simulink model "LQR1"  (R2020a)
settings: Solver=VariableStepAuto  StartTime=0.0  StopTime=300  RelTol=1e-3
values from neighbouring files (symbols this model uses):
  A = zeros(n_states)    [RIP.m]
  B = zeros(n_states,n_inputs)    [RIP.m]
  Ki = K_d_Int(:,1)    [RIP.m]
  Ks = K_d_Int(:,2:end)    [RIP.m]
  n_inputs = 1    [RIP.m]
  n_states = 4    [RIP.m]
  Ts = 1/200    (= 0.005)    [RIP.m]
libraries: dspsrcs4 x1
settings Model: Creator=user  LastModifiedBy=user

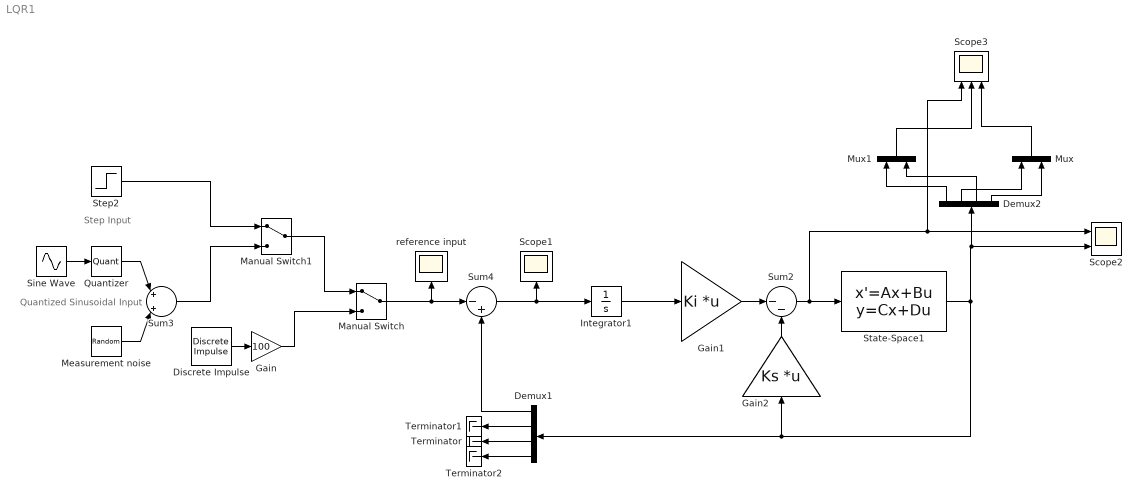
== system LQR1 ==
  note: Quantized Sinusoidal Input
  note: Step Input
  Demux1 : Demux
  Demux2 : Demux
  Discrete Impulse : dspsrcs4/Discrete  Impulse  Delay=0  SampleTime=0.01  FrameSample=1  OutputFrames=off  dataType=double  isSigned=on  wordLen=16  udDataType=sfix(16)  fracBitsMode=Best precision  numFracBits=15  OutDataTypeStr=double  LastOutDataTypeStr=double
  Gain : Gain  Gain=100
  Gain1 : Gain  Gain=Ki  Multiplication=Matrix(K*u)
  Gain2 : Gain  Gain=Ks  Multiplication=Matrix(K*u)
  Integrator1 : Integrator
  Manual Switch : ManualSwitch
  Manual Switch1 : ManualSwitch
  Measurement noise : RandomNumber  Variance=0.0000001  SampleTime=Ts
  Mux : Mux  Inputs=2
  Mux1 : Mux  Inputs=2
  Quantizer : Quantizer  QuantizationInterval=2^(-12)
  Scope1 : Scope
  Scope2 : Scope  NumInputPorts=2
  Scope3 : Scope  NumInputPorts=3
  Sine Wave : Sin  Amplitude=pi/4  Frequency=0.2  SampleTime=Ts
  State-Space1 : StateSpace  A=A  B=B  C=eye(n_states)  D=zeros(n_states,n_inputs)  InitialCondition=0
  Step2 : Step  After=pi/3  SampleTime=Ts
  Sum2 : Sum  Inputs=|--
  Sum3 : Sum  Inputs=|+|+|
  Sum4 : Sum  Inputs=|-+
  Terminator : Terminator
  Terminator1 : Terminator
  Terminator2 : Terminator
  reference input : Scope
  wires:
  State-Space1/1 -> Demux2/1, Scope2/2, Gain2/1, Demux1/1
  Demux1/1 -> Sum4/2
  Integrator1/1 -> Gain1/1
  Demux1/3 -> Terminator/1
  Sum2/1 -> Scope3/1, Scope2/1, State-Space1/1
  Gain2/1 -> Sum2/2
  Gain1/1 -> Sum2/1
  Demux1/2 -> Terminator1/1
  Demux1/4 -> Terminator2/1
  Manual Switch/1 -> reference input/1, Sum4/1
  Discrete Impulse/1 -> Gain/1
  Sine Wave/1 -> Quantizer/1
  Quantizer/1 -> Sum3/1
  Measurement noise/1 -> Sum3/2
  Step2/1 -> Manual Switch1/1
  Manual Switch1/1 -> Manual Switch/1
  Sum3/1 -> Manual Switch1/2
  Sum4/1 -> Integrator1/1, Scope1/1
  Gain/1 -> Manual Switch/2
  Demux2/1 -> Mux1/1
  Demux2/3 -> Mux1/2
  Demux2/2 -> Mux/1
  Demux2/4 -> Mux/2
  Mux1/1 -> Scope3/2
  Mux/1 -> Scope3/3
